simulink model "Vorlage_Gesamtanlage"  (R2022a)
settings: Solver=ode5  StartTime=0.0  StopTime=200  FixedStep=0.01  MaxStep=1  MinStep=0.005  RelTol=1e-3  AbsTol=10  EnableMultiTasking=on
values from neighbouring files (symbols this model uses):
  A = 5    [Parameter.m]
  Flaschengroesse = 10    [Parameter.m]
  I = 0.5    [Parameter.m]
  igetr = 1080    [Parameter.m]
  K = 8    [Parameter.m]
  MaxFlaschen = 25    [Parameter.m]
  MRK = 1    [Parameter.m]
  numA = 0    [Parameter.m]
  PassSilo1 = 1    [Parameter.m]
  PassSilo2 = 1    [Parameter.m]
  PHI = 0.001    [Parameter.m]
  Ra = 40    [Parameter.m]
  SizeSilo1 = 15    [Parameter.m]
  SizeSilo2 = 15    [Parameter.m]
  U = 24    [Parameter.m]
  v_band_abfuhr_set = 2    [Parameter.m]
  v_band_arbeit_set = 30    [Parameter.m]
  v_band_zufuhr_set = 10    [Parameter.m]
  v_umsetzer_greifer_set = 400    [Parameter.m]
  v_umsetzer_set = 80    [Parameter.m]
  v_ve1_set = 400    [Parameter.m]
  v_ve2_set = 400    [Parameter.m]
undefined symbols (not defined in the file or in its folder): Limits
libraries: simulink x94
(part 1 of 3)
settings Model: Creator=merz  LastModifiedBy=yufu
settings SolverCC: AutoScaleAbsTol=off  AlgebraicLoopSolver=TrustRegion
settings DataIOCC: LimitDataPoints=on  SaveFormat=Array  SignalLoggingSaveFormat=ModelDataLogs  ReturnWorkspaceOutputs=off  SignalLoggingName=sigsOut
settings OptimizationCC: ExpressionDepthLimit=2147483647  InitFltsAndDblsToZero=on  LifeSpan=inf
settings DebuggingCC: AlgebraicLoopMsg=none  SaveWithParameterizedLinksMsg=none  UnderspecifiedInitializationDetection=Classic  MergeDetectMultiDrivingBlocksExec=none  SignalResolutionControl=TryResolveAllWithWarning  MultiTaskDSMMsg=warning  MultiTaskCondExecSysMsg=none  FcnCallInpInsideContextMsg=warning  UnconnectedInputMsg=warning  UnconnectedOutputMsg=warning  UnconnectedLineMsg=warning  StateNameClashWarn=warning  SFUnexpectedBacktrackingDiag=warning  SFNoUnconditionalDefaultTransitionDiag=warning  SFMachineParentedDataDiag=warning  ArithmeticOperatorsInVariantConditions=warning
settings HardwareCC: ProdBitPerPointer=32  ProdBitPerSizeT=32  ProdBitPerPtrDiffT=32  ProdLargestAtomicFloat=None  ProdIntDivRoundTo=Undefined  ProdEndianess=Unspecified  ProdWordSize=32  ProdHWDeviceType=32-bit Generic  TargetUnknown=on
settings ModelReferenceCC: PropagateSignalLabelsOutOfModel=off
settings SFSimCC: SimUseLocalCustomCode=off  SimParseCustomCode=off  CustomCodeUndefinedFunction=UseInterfaceOnly
settings RTWCC: RTWUseLocalCustomCode=off
settings CodeAppCC: StateflowObjectComments=on
settings GRTTargetCC: TargetFcnLib=ansi_tfl_tmw.mat  TargetLangStandard=C89/C90 (ANSI)  ModelReferenceCompliant=off  CombineOutputUpdateFcns=off  MatFileLogging=off  GRTInterface=on
settings ConfigComp: CovMetricSettings=dw  CovSaveCumulativeToWorkspaceVar=on  CovSaveSingleToWorkspaceVar=on  CovExternalEMLEnable=off  CovSFcnEnable=off

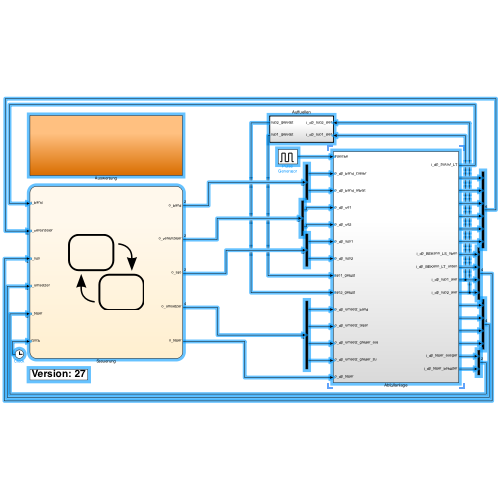
[thumbnail: Simulink's stored preview of the top-level diagram]
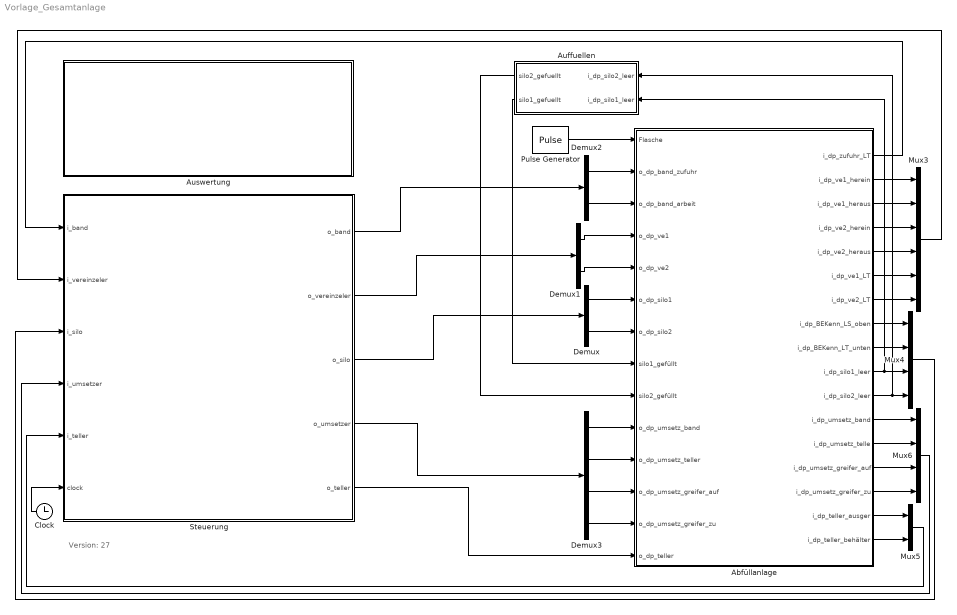
== system Vorlage_Gesamtanlage ==
  note: Version: 27
  Abfüllanlage : Subsystem
  Auffuellen : Subsystem  TreatAsAtomicUnit=on
  Auswertung : Subsystem
  Clock : Clock
  Demux : Demux  Outputs=2
      settings: DisplayOption=none
  Demux1 : Demux  Outputs=2
      settings: DisplayOption=none
  Demux2 : Demux  Outputs=2
      settings: DisplayOption=none
  Demux3 : Demux
      settings: DisplayOption=none
  Mux3 : Mux  Inputs=6
  Mux4 : Mux
  Mux5 : Mux  Inputs=2
  Mux6 : Mux
  Pulse Generator : DiscretePulseGenerator  PulseType=Time based  Period=5  PulseWidth=10  PhaseDelay=2
  Steuerung : Stateflow chart  TreatAsAtomicUnit=on
  wires:
  Steuerung/1(o_band) -> Demux2/1
  Steuerung/4(o_umsetzer) -> Demux3/1
  Steuerung/3(o_silo) -> Demux/1
  Steuerung/2(o_vereinzeler) -> Demux1/1
  Abfüllanlage/5(i_dp_ve2_heraus) -> Mux3/4
  Abfüllanlage/6(i_dp_ve1_LT) -> Mux3/5
  Abfüllanlage/7(i_dp_ve2_LT) -> Mux3/6
  Mux3/1 -> Steuerung/2(i_vereinzeler)
  Abfüllanlage/11(i_dp_silo2_leer) -> Auffuellen/1(i_dp_silo2_leer), Mux4/4
  Abfüllanlage/10(i_dp_silo1_leer) -> Mux4/3, Auffuellen/2(i_dp_silo1_leer)
  Abfüllanlage/8(i_dp_BEKenn_LS_oben) -> Mux4/1
  Abfüllanlage/16(i_dp_teller_ausger) -> Mux5/1
  Abfüllanlage/17(i_dp_teller_behälter) -> Mux5/2
  Mux5/1 -> Steuerung/5(i_teller)
  Abfüllanlage/1(i_dp_zufuhr_LT) -> Steuerung/1(i_band)
  Mux6/1 -> Steuerung/4(i_umsetzer)
  Demux/1 -> Abfüllanlage/6(o_dp_silo1)
  Demux/2 -> Abfüllanlage/7(o_dp_silo2)
  Demux1/1 -> Abfüllanlage/4(o_dp_ve1)
  Demux1/2 -> Abfüllanlage/5(o_dp_ve2)
  Demux2/1 -> Abfüllanlage/2(o_dp_band_zufuhr)
  Demux2/2 -> Abfüllanlage/3(o_dp_band_arbeit)
  Pulse Generator/1 -> Abfüllanlage/1(Flasche)
  Mux4/1 -> Steuerung/3(i_silo)
  Abfüllanlage/3(i_dp_ve1_heraus) -> Mux3/2
  Abfüllanlage/2(i_dp_ve1_herein) -> Mux3/1
  Abfüllanlage/4(i_dp_ve2_herein) -> Mux3/3
  Auffuellen/2(silo1_gefuellt) -> Abfüllanlage/8(silo1_gefüllt)
  Auffuellen/1(silo2_gefuellt) -> Abfüllanlage/9(silo2_gefüllt)
  Abfüllanlage/12(i_dp_umsetz_band) -> Mux6/1
  Abfüllanlage/13(i_dp_umsetz_telle) -> Mux6/2
  Abfüllanlage/14(i_dp_umsetz_greifer_auf) -> Mux6/3
  Abfüllanlage/15(i_dp_umsetz_greifer_zu) -> Mux6/4
  Demux3/1 -> Abfüllanlage/10(o_dp_umsetz_band)
  Demux3/2 -> Abfüllanlage/11(o_dp_umsetz_teller)
  Demux3/3 -> Abfüllanlage/12(o_dp_umsetz_greifer_auf)
  Demux3/4 -> Abfüllanlage/13(o_dp_umsetz_greifer_zu)
  Steuerung/5(o_teller) -> Abfüllanlage/14(o_dp_teller)
  Clock/1 -> Steuerung/6(clock)
  Abfüllanlage/9(i_dp_BEKenn_LT_unten) -> Mux4/2

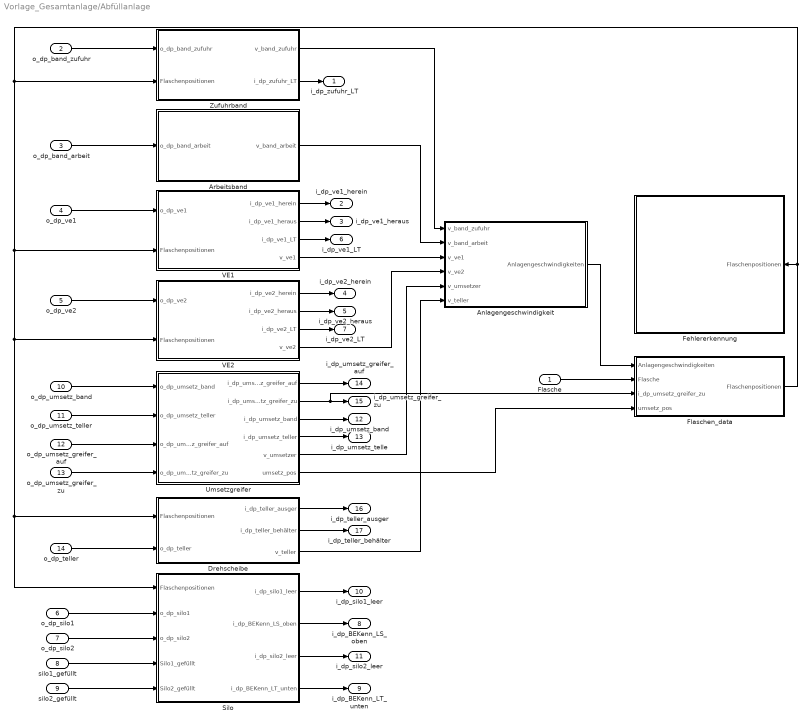
== system Vorlage_Gesamtanlage/Abfüllanlage ==
  Flasche : Inport
  o_dp_band_zufuhr : Inport  Port=2  OutDataTypeStr=double
  o_dp_band_arbeit : Inport  Port=3  OutDataTypeStr=double
  o_dp_ve1 : Inport  Port=4  OutDataTypeStr=double
  o_dp_ve2 : Inport  Port=5  OutDataTypeStr=double
  o_dp_silo1 : Inport  Port=6  OutDataTypeStr=double
  o_dp_silo2 : Inport  Port=7  OutDataTypeStr=double
  silo1_gefüllt : Inport  Port=8  OutDataTypeStr=double
  silo2_gefüllt : Inport  Port=9  OutDataTypeStr=double
  o_dp_umsetz_band : Inport  Port=10  OutDataTypeStr=double
  o_dp_umsetz_teller : Inport  Port=11  OutDataTypeStr=double
  o_dp_umsetz_greifer_auf : Inport  Port=12  OutDataTypeStr=double
  o_dp_umsetz_greifer_zu : Inport  Port=13  OutDataTypeStr=double
  o_dp_teller : Inport  Port=14  OutDataTypeStr=double
  Anlagengeschwindigkeit : Subsystem
  Arbeitsband : Subsystem
  Drehscheibe : Subsystem
  Fehlererkennung : Subsystem
  Flaschen_data : Subsystem
  Silo : Subsystem
  Umsetzgreifer : Subsystem
  VE1 : Subsystem
  VE2 : Subsystem
  Zufuhrband : Subsystem
  i_dp_zufuhr_LT : Outport  OutDataTypeStr=boolean
  i_dp_ve1_herein : Outport  Port=2  OutDataTypeStr=boolean
  i_dp_ve1_heraus : Outport  Port=3  OutDataTypeStr=boolean
  i_dp_ve2_herein : Outport  Port=4  OutDataTypeStr=boolean
  i_dp_ve2_heraus : Outport  Port=5  OutDataTypeStr=boolean
  i_dp_ve1_LT : Outport  Port=6  OutDataTypeStr=boolean
  i_dp_ve2_LT : Outport  Port=7  OutDataTypeStr=boolean
  i_dp_BEKenn_LS_oben : Outport  Port=8  OutDataTypeStr=boolean
  i_dp_BEKenn_LT_unten : Outport  Port=9  OutDataTypeStr=boolean
  i_dp_silo1_leer : Outport  Port=10  OutDataTypeStr=boolean
  i_dp_silo2_leer : Outport  Port=11  OutDataTypeStr=boolean
  i_dp_umsetz_band : Outport  Port=12  OutDataTypeStr=boolean
  i_dp_umsetz_telle : Outport  Port=13  OutDataTypeStr=boolean
  i_dp_umsetz_greifer_auf : Outport  Port=14  OutDataTypeStr=boolean
  i_dp_umsetz_greifer_zu : Outport  Port=15  OutDataTypeStr=boolean
  i_dp_teller_ausger : Outport  Port=16  OutDataTypeStr=boolean
  i_dp_teller_behälter : Outport  Port=17  OutDataTypeStr=boolean
  wires:
  Zufuhrband/1(v_band_zufuhr) -> Anlagengeschwindigkeit/1(v_band_zufuhr)
  VE1/4(v_ve1) -> Anlagengeschwindigkeit/3(v_ve1)
  Umsetzgreifer/5(v_umsetzer) -> Anlagengeschwindigkeit/5(v_umsetzer)
  Drehscheibe/3(v_teller) -> Anlagengeschwindigkeit/6(v_teller)
  Flaschen_data/1(Flaschenpositionen) -> Zufuhrband/2(Flaschenpositionen), VE1/2(Flaschenpositionen), VE2/2(Flaschenpositionen), Silo/1(Flaschenpositionen), Drehscheibe/1(Flaschenpositionen), Fehlererkennung/1(Flaschenpositionen)
  o_dp_band_zufuhr/1 -> Zufuhrband/1(o_dp_band_zufuhr)
  Zufuhrband/2(i_dp_zufuhr_LT) -> i_dp_zufuhr_LT/1
  o_dp_band_arbeit/1 -> Arbeitsband/1(o_dp_band_arbeit)
  VE1/1(i_dp_ve1_herein) -> i_dp_ve1_herein/1
  o_dp_ve1/1 -> VE1/1(o_dp_ve1)
  Silo/1(i_dp_silo1_leer) -> i_dp_silo1_leer/1
  VE1/2(i_dp_ve1_heraus) -> i_dp_ve1_heraus/1
  Silo/2(i_dp_BEKenn_LS_oben) -> i_dp_BEKenn_LS_oben/1
  VE1/3(i_dp_ve1_LT) -> i_dp_ve1_LT/1
  Silo/3(i_dp_silo2_leer) -> i_dp_silo2_leer/1
  Silo/4(i_dp_BEKenn_LT_unten) -> i_dp_BEKenn_LT_unten/1
  Umsetzgreifer/1(i_dp_umsetz_greifer_auf) -> i_dp_umsetz_greifer_auf/1
  o_dp_umsetz_band/1 -> Umsetzgreifer/1(o_dp_umsetz_band)
  o_dp_umsetz_teller/1 -> Umsetzgreifer/2(o_dp_umsetz_teller)
  Umsetzgreifer/3(i_dp_umsetz_band) -> i_dp_umsetz_band/1
  o_dp_umsetz_greifer_auf/1 -> Umsetzgreifer/3(o_dp_umsetz_greifer_auf)
  Umsetzgreifer/4(i_dp_umsetz_teller) -> i_dp_umsetz_telle/1
  o_dp_umsetz_greifer_zu/1 -> Umsetzgreifer/4(o_dp_umsetz_greifer_zu)
  Drehscheibe/1(i_dp_teller_ausger) -> i_dp_teller_ausger/1
  o_dp_teller/1 -> Drehscheibe/2(o_dp_teller)
  Drehscheibe/2(i_dp_teller_behälter) -> i_dp_teller_behälter/1
  o_dp_silo1/1 -> Silo/2(o_dp_silo1)
  o_dp_silo2/1 -> Silo/3(o_dp_silo2)
  silo2_gefüllt/1 -> Silo/5(Silo2_gefüllt)
  silo1_gefüllt/1 -> Silo/4(Silo1_gefüllt)
  Flasche/1 -> Flaschen_data/2(Flasche)
  Anlagengeschwindigkeit/1(Anlagengeschwindigkeiten) -> Flaschen_data/1(Anlagengeschwindigkeiten)
  VE2/2(i_dp_ve2_heraus) -> i_dp_ve2_heraus/1
  VE2/1(i_dp_ve2_herein) -> i_dp_ve2_herein/1
  VE2/3(i_dp_ve2_LT) -> i_dp_ve2_LT/1
  VE2/4(v_ve2) -> Anlagengeschwindigkeit/4(v_ve2)
  o_dp_ve2/1 -> VE2/1(o_dp_ve2)
  Umsetzgreifer/2(i_dp_umsetz_greifer_zu) -> i_dp_umsetz_greifer_zu/1, Flaschen_data/3(i_dp_umsetz_greifer_zu)
  Arbeitsband/1(v_band_arbeit) -> Anlagengeschwindigkeit/2(v_band_arbeit)
  Umsetzgreifer/6(umsetz_pos) -> Flaschen_data/4(umsetz_pos)

== system Vorlage_Gesamtanlage/Auffuellen ==
  i_dp_silo2_leer : Inport
  i_dp_silo1_leer : Inport  Port=2
  Data Type Conversion : DataTypeConversion  OutDataTypeStr=double  SaturateOnIntegerOverflow=off  RndMeth=Floor
  Data Type Conversion1 : DataTypeConversion  OutDataTypeStr=double  SaturateOnIntegerOverflow=off  RndMeth=Floor
  Transport Delay : TransportDelay  DelayTime=10
  Transport Delay1 : TransportDelay  DelayTime=10
  silo2_gefuellt : Outport
  silo1_gefuellt : Outport  Port=2
  wires:
  i_dp_silo1_leer/1 -> Data Type Conversion/1
  Transport Delay/1 -> silo1_gefuellt/1
  i_dp_silo2_leer/1 -> Data Type Conversion1/1
  Transport Delay1/1 -> silo2_gefuellt/1
  Data Type Conversion/1 -> Transport Delay/1
  Data Type Conversion1/1 -> Transport Delay1/1

== system Vorlage_Gesamtanlage/Auswertung ==
  Arbeitsband : Subsystem
  Drehscheibe : Subsystem
  Flaschen_data : Subsystem
  Gesamt : Subsystem
  Silo : Subsystem
  Umsetzgreifer : Subsystem
  Vereinzelner 1 : Subsystem
  Vereinzelner 2 : Subsystem
  Zufuhrband : Subsystem

== system Vorlage_Gesamtanlage/Abfüllanlage/Anlagengeschwindigkeit ==
  v_band_zufuhr : Inport
  v_band_arbeit : Inport  Port=2
  v_ve1 : Inport  Port=3
  v_ve2 : Inport  Port=4
  v_umsetzer : Inport  Port=5
  v_teller : Inport  Port=6
  Gain : Gain  Gain=3  SaturateOnIntegerOverflow=on  OutDataTypeStr=Inherit: Same as input  ParamDataTypeStr=Inherit: Same as input
  Mux : Mux  Inputs=10
  Wartestellung : Constant  Value=0
  v_band_abfuhr : Constant  Value=v_band_abfuhr_set
  Anlagengeschwindigkeiten : Outport
  wires:
  v_band_arbeit/1 -> Gain/1, Mux/3
  v_umsetzer/1 -> Mux/8, Mux/6
  Mux/1 -> Anlagengeschwindigkeiten/1
  v_band_abfuhr/1 -> Mux/10
  v_ve2/1 -> Mux/9
  v_teller/1 -> Mux/7
  Gain/1 -> Mux/5
  v_ve1/1 -> Mux/4
  v_band_zufuhr/1 -> Mux/2
  Wartestellung/1 -> Mux/1

== system Vorlage_Gesamtanlage/Abfüllanlage/Arbeitsband ==
  o_dp_band_arbeit : Inport
  Gain : Gain  Gain=v_band_arbeit_set  OutDataTypeStr=Inherit: Inherit via back propagation  SaturateOnIntegerOverflow=on  ParamDataTypeStr=Inherit: Same as input
  v_band_arbeit : Outport  OutDataTypeStr=double
  tag scope: o_dp_band_arbeit=global, v_band_arbeit=global
  wires:
  o_dp_band_arbeit/1 -> Gain/1, [o_dp_band_arbeit]  "o_dp_band_arbeit"
  Gain/1 -> v_band_arbeit/1, [v_band_arbeit]  "v_band_arbeit"

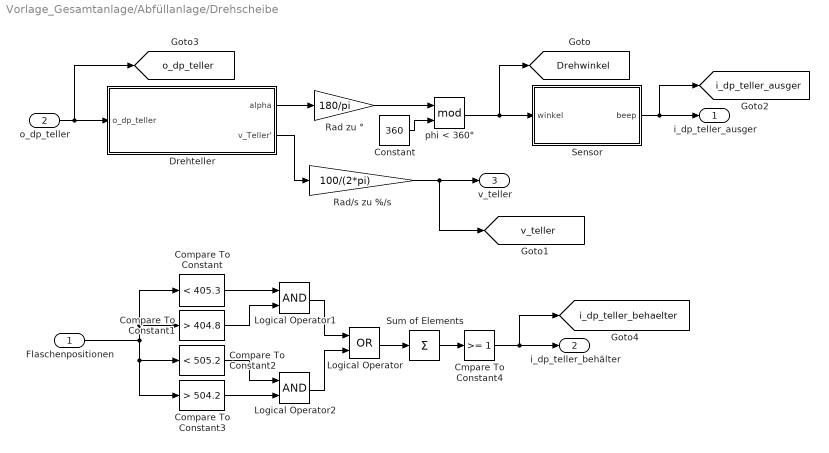
== system Vorlage_Gesamtanlage/Abfüllanlage/Drehscheibe ==
  Flaschenpositionen : Inport
  o_dp_teller : Inport  Port=2
  Cmpare To Constant4 : simulink/Logic and Bit Operations/Compare To Constant  relop=>=  const=1  OutDataTypeStr=boolean  ZeroCross=off
  Compare To Constant : simulink/Logic and Bit Operations/Compare To Constant  relop=<  const=405.3  OutDataTypeStr=boolean  ZeroCross=off
  Compare To Constant1 : simulink/Logic and Bit Operations/Compare To Constant  relop=>  const=404.8  OutDataTypeStr=boolean  ZeroCross=off
  Compare To Constant2 : simulink/Logic and Bit Operations/Compare To Constant  relop=<  const=505.2  OutDataTypeStr=boolean  ZeroCross=off
  Compare To Constant3 : simulink/Logic and Bit Operations/Compare To Constant  relop=>  const=504.2  OutDataTypeStr=boolean  ZeroCross=off
  Constant : Constant  Value=360
  Drehteller : Subsystem
  Logical Operator : Logic  Operator=OR  AllPortsSameDT=off  OutDataTypeStr=boolean
  Logical Operator1 : Logic  AllPortsSameDT=off  OutDataTypeStr=boolean
  Logical Operator2 : Logic  AllPortsSameDT=off  OutDataTypeStr=boolean
  Rad zu ° : Gain  Gain=180/pi  SaturateOnIntegerOverflow=on  OutDataTypeStr=Inherit: Same as input  ParamDataTypeStr=Inherit: Same as input
  Rad/s zu %/s : Gain  Gain=100/(2*pi)  SaturateOnIntegerOverflow=on  OutDataTypeStr=Inherit: Same as input  ParamDataTypeStr=Inherit: Same as input
  Sensor : Stateflow chart  TreatAsAtomicUnit=on
  Sum of Elements : Sum  Inputs=+
  phi < 360° : Math  Operator=mod  SignedPower=on
  i_dp_teller_ausger : Outport  OutDataTypeStr=boolean
  i_dp_teller_behälter : Outport  Port=2  OutDataTypeStr=boolean
  v_teller : Outport  Port=3  OutDataTypeStr=double
  tag scope: Drehwinkel=global, i_dp_teller_ausger=global, i_dp_teller_behaelter=global, o_dp_teller=global, v_teller=global
  wires:
  Sensor/1(beep) -> i_dp_teller_ausger/1, [i_dp_teller_ausger]
  phi < 360°/1 -> [Drehwinkel], Sensor/1(winkel)
  Rad zu °/1 -> phi < 360°/1
  Rad/s zu %/s/1 -> v_teller/1, [v_teller]
  Constant/1 -> phi < 360°/2
  o_dp_teller/1 -> Drehteller/1(o_dp_teller), [o_dp_teller]
  Drehteller/1(alpha) -> Rad zu °/1
  Drehteller/2(v_Teller') -> Rad/s zu %/s/1
  Logical Operator/1 -> Sum of Elements/1
  Compare To Constant/1 -> Logical Operator1/1
  Compare To Constant1/1 -> Logical Operator1/2
  Logical Operator1/1 -> Logical Operator/1
  Compare To Constant3/1 -> Logical Operator2/2
  Compare To Constant2/1 -> Logical Operator2/1
  Logical Operator2/1 -> Logical Operator/2
  Sum of Elements/1 -> Cmpare To Constant4/1
  Flaschenpositionen/1 -> Compare To Constant/1, Compare To Constant1/1, Compare To Constant3/1, Compare To Constant2/1
  Cmpare To Constant4/1 -> i_dp_teller_behälter/1, [i_dp_teller_behaelter]

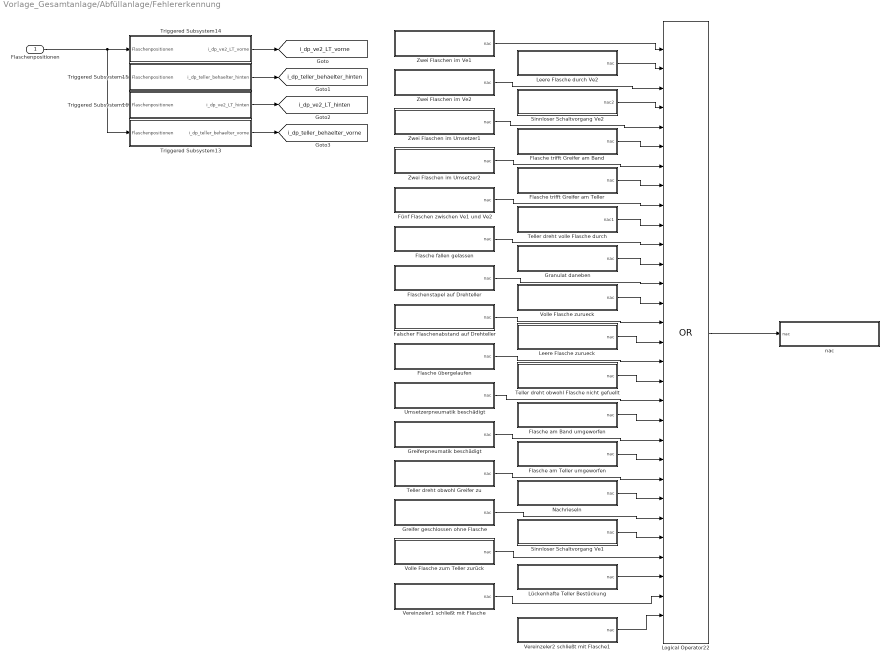
== system Vorlage_Gesamtanlage/Abfüllanlage/Fehlererkennung ==
  Flaschenpositionen : Inport
  Falscher Flaschenabstand auf Drehteller : Subsystem
  Flasche am Band umgeworfen : Subsystem
  Flasche am Teller umgeworfen : Subsystem
  Flasche fallen gelassen : Subsystem
  Flasche trifft Greifer am Band : Subsystem
  Flasche trifft Greifer am Teller : Subsystem
  Flasche übergelaufen : Subsystem
  Flaschenstapel auf Drehteller : Subsystem
  Fünf Flaschen zwischen Ve1 und Ve2 : Subsystem
  Granulat daneben : Subsystem
  Greifer geschlossen ohne Flasche : Subsystem
  Greiferpneumatik beschädigt : Subsystem
  Leere Flasche durch Ve2 : Subsystem
  Leere Flasche zurueck : Subsystem
  Logical Operator22 : Logic  Operator=OR  Inputs=30  AllPortsSameDT=off  OutDataTypeStr=boolean
  Lückenhafte Teller Bestückung : Subsystem
  Nachrieseln : Subsystem
  Sinnloser Schaltvorgang Ve1 : Subsystem
  Sinnloser Schaltvorgang Ve2 : Subsystem
  Teller dreht obwohl Flasche nicht gefuellt : Subsystem
  Teller dreht obwohl Greifer zu : Subsystem
  Teller dreht volle Flasche durch : Subsystem
  Triggered Subsystem13 : Subsystem  TreatAsAtomicUnit=on
  Triggered Subsystem14 : Subsystem  TreatAsAtomicUnit=on
  Triggered Subsystem15 : Subsystem  TreatAsAtomicUnit=on
  Triggered Subsystem16 : Subsystem  TreatAsAtomicUnit=on
  Umsetzerpneumatik beschädigt : Subsystem
  Vereinzeler1 schließt mit Flasche : Subsystem
  Vereinzeler2 schließt mit Flasche1 : Subsystem
  Volle Flasche zum Teller zurück : Subsystem
  Volle Flasche zurueck : Subsystem
  Zwei Flaschen im Umsetzer1 : Subsystem
  Zwei Flaschen im Umsetzer2 : Subsystem
  Zwei Flaschen im Ve1 : Subsystem
  Zwei Flaschen im Ve2 : Subsystem
  nac : Subsystem
  tag scope: i_dp_teller_behaelter_hinten=global, i_dp_teller_behaelter_vorne=global, i_dp_ve2_LT_hinten=global, i_dp_ve2_LT_vorne=global
  wires:
  Leere Flasche durch Ve2/1(nac) -> Logical Operator22/2
  Sinnloser Schaltvorgang Ve2/1(nac2) -> Logical Operator22/4
  Flasche trifft Greifer am Band/1(nac) -> Logical Operator22/6
  Flasche trifft Greifer am Teller/1(nac) -> Logical Operator22/8
  Teller dreht volle Flasche durch/1(nac1) -> Logical Operator22/10
  Granulat daneben/1(nac) -> Logical Operator22/12
  Flaschenstapel auf Drehteller/1(nac) -> Logical Operator22/13
  Volle Flasche zurueck/1(nac) -> Logical Operator22/14
  Flasche übergelaufen/1(nac) -> Logical Operator22/17
  Leere Flasche zurueck/1(nac) -> Logical Operator22/16
  Umsetzerpneumatik beschädigt/1(nac) -> Logical Operator22/19
  Teller dreht obwohl Flasche nicht gefuellt/1(nac) -> Logical Operator22/18
  Greiferpneumatik beschädigt/1(nac) -> Logical Operator22/21
  Flasche am Band umgeworfen/1(nac) -> Logical Operator22/20
  Flasche am Teller umgeworfen/1(nac) -> Logical Operator22/22
  Teller dreht obwohl Greifer zu/1(nac) -> Logical Operator22/23
  Falscher Flaschenabstand auf Drehteller/1(nac) -> Logical Operator22/15
  Flasche fallen gelassen/1(nac) -> Logical Operator22/11
  Fünf Flaschen zwischen Ve1 und Ve2/1(nac) -> Logical Operator22/9
  Zwei Flaschen im Umsetzer2/1(nac) -> Logical Operator22/7
  Zwei Flaschen im Umsetzer1/1(nac) -> Logical Operator22/5
  Zwei Flaschen im Ve2/1(nac) -> Logical Operator22/3
  Zwei Flaschen im Ve1/1(nac) -> Logical Operator22/1
  Triggered Subsystem14/1(i_dp_ve2_LT_vorne) -> [i_dp_ve2_LT_vorne]
  Triggered Subsystem15/1(i_dp_teller_behaelter_hinten) -> [i_dp_teller_behaelter_hinten]
  Triggered Subsystem16/1(i_dp_ve2_LT_hinten) -> [i_dp_ve2_LT_hinten]
  Triggered Subsystem13/1(i_dp_teller_behaelter_vorne) -> [i_dp_teller_behaelter_vorne]
  Flaschenpositionen/1 -> Triggered Subsystem14/1(Flaschenpositionen), Triggered Subsystem15/1(Flaschenpositionen), Triggered Subsystem16/1(Flaschenpositionen), Triggered Subsystem13/1(Flaschenpositionen)
  Nachrieseln/1(nac) -> Logical Operator22/24
  Greifer geschlossen ohne Flasche/1(nac) -> Logical Operator22/25
  Sinnloser Schaltvorgang Ve1/1(nac) -> Logical Operator22/26
  Volle Flasche zum Teller zurück/1(nac) -> Logical Operator22/27
  Lückenhafte Teller Bestückung/1(nac) -> Logical Operator22/28
  Vereinzeler1 schließt mit Flasche/1(nac) -> Logical Operator22/29
  Vereinzeler2 schließt mit Flasche1/1(nac) -> Logical Operator22/30
  Logical Operator22/1 -> nac/1(nac)

== system Vorlage_Gesamtanlage/Abfüllanlage/Flaschen_data ==
  Anlagengeschwindigkeiten : Inport
  Flasche : Inport  Port=2
  i_dp_umsetz_greifer_zu : Inport  Port=3
  umsetz_pos : Inport  Port=4
  Constant : Constant  Value=[0.01 101 201 205 305 405 505 605 610 inf]
  Flaschengeschwindigkeiten : Subsystem
  Flaschenstarter : Subsystem
  "v -> x" : Subsystem
  Flaschenpositionen : Outport
  tag scope: Flaschengeschwindigkeiten=global, Flaschenpositionen=global
  wires:
  Flasche/1 -> Flaschenstarter/2(Flasche)
  Flaschengeschwindigkeiten/1(Flaschengeschwindigkeiten) -> [Flaschengeschwindigkeiten], "v -> x"/1(Flaschengeschwindigkeiten)
  Anlagengeschwindigkeiten/1 -> Flaschengeschwindigkeiten/1(Anlagengeschwindigkeiten)
  Flaschenstarter/1(Flaschenpositionen mit Starter) -> Flaschengeschwindigkeiten/3(Flaschenpositionen)
  i_dp_umsetz_greifer_zu/1 -> Flaschengeschwindigkeiten/2(i_dp_umsetz_greifer_zu)
  umsetz_pos/1 -> Flaschengeschwindigkeiten/4(umsetz_pos)
  "v -> x"/1(Flaschenpositionen) -> Flaschenpositionen/1, [Flaschenpositionen], Flaschenstarter/1(Flaschenpositionen)
  Flaschengeschwindigkeiten/2(Anlagenpositionen) -> "v -> x"/2(Anlagenpositionen)
  Constant/1 -> "v -> x"/3(Anlagenlimits)

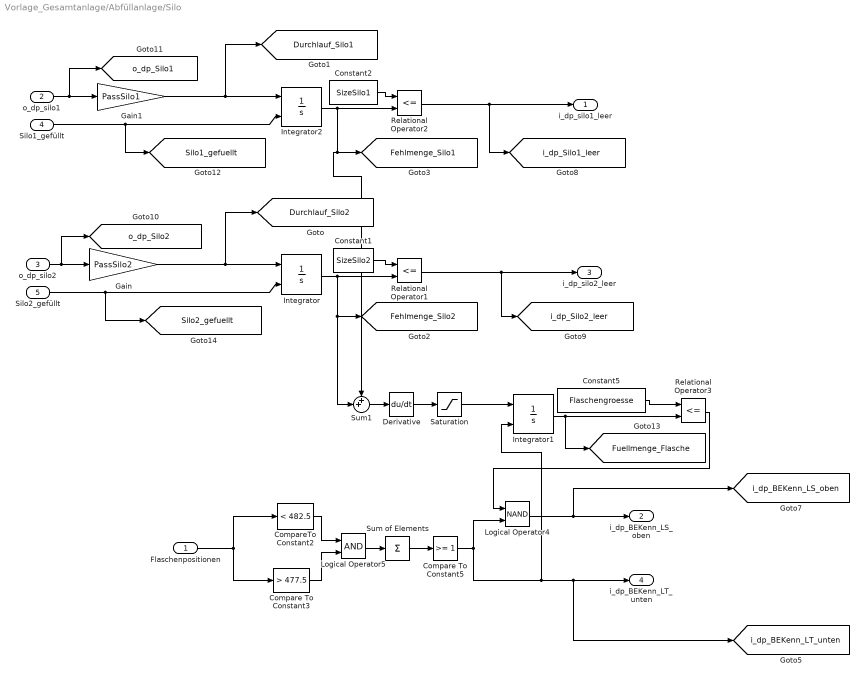
== system Vorlage_Gesamtanlage/Abfüllanlage/Silo ==
  Flaschenpositionen : Inport
  o_dp_silo1 : Inport  Port=2
  o_dp_silo2 : Inport  Port=3
  Silo1_gefüllt : Inport  Port=4
  Silo2_gefüllt : Inport  Port=5
  Compare To Constant3 : simulink/Logic and Bit Operations/Compare To Constant  relop=>  const=477.5  OutDataTypeStr=boolean  ZeroCross=off
  Compare To Constant5 : simulink/Logic and Bit Operations/Compare To Constant  relop=>=  const=1  OutDataTypeStr=boolean  ZeroCross=off
  CompareTo Constant2 : simulink/Logic and Bit Operations/Compare To Constant  relop=<  const=482.5  OutDataTypeStr=boolean  ZeroCross=off
  Constant1 : Constant  Value=SizeSilo2
  Constant2 : Constant  Value=SizeSilo1
  Constant5 : Constant  Value=Flaschengroesse
  Derivative : Derivative
  Gain : Gain  Gain=PassSilo2  SaturateOnIntegerOverflow=on  OutDataTypeStr=Inherit: Same as input  ParamDataTypeStr=Inherit: Same as input
  Gain1 : Gain  Gain=PassSilo1  SaturateOnIntegerOverflow=on  OutDataTypeStr=Inherit: Same as input  ParamDataTypeStr=Inherit: Same as input
  Integrator : Integrator  ExternalReset=rising  LimitOutput=on  UpperSaturationLimit=SizeSilo2  LowerSaturationLimit=0
  Integrator1 : Integrator  ExternalReset=falling  LimitOutput=on  LowerSaturationLimit=0
  Integrator2 : Integrator  ExternalReset=rising  LimitOutput=on  UpperSaturationLimit=SizeSilo1  LowerSaturationLimit=0
  Logical Operator4 : Logic  Operator=NAND  AllPortsSameDT=off  OutDataTypeStr=boolean
  Logical Operator5 : Logic  AllPortsSameDT=off  OutDataTypeStr=boolean
  Relational Operator1 : RelationalOperator  Operator=<=  InputSameDT=off
  Relational Operator2 : RelationalOperator  Operator=<=  InputSameDT=off
  Relational Operator3 : RelationalOperator  Operator=<=  InputSameDT=off
  Saturation : Saturate  UpperLimit=inf  LowerLimit=0
  Sum of Elements : Sum  Inputs=+
  Sum1 : Sum  Inputs=++|  SaturateOnIntegerOverflow=on
  i_dp_silo1_leer : Outport  OutDataTypeStr=boolean
  i_dp_BEKenn_LS_oben : Outport  Port=2  OutDataTypeStr=boolean
  i_dp_silo2_leer : Outport  Port=3  OutDataTypeStr=boolean
  i_dp_BEKenn_LT_unten : Outport  Port=4  OutDataTypeStr=boolean
  tag scope: Durchlauf_Silo1=global, Durchlauf_Silo2=global, Fehlmenge_Silo1=global, Fehlmenge_Silo2=global, Fuellmenge_Flasche=global, Silo1_gefuellt=global, Silo2_gefuellt=global, i_dp_BEKenn_LS_oben=global, i_dp_BEKenn_LT_unten=global, i_dp_Silo1_leer=global, i_dp_Silo2_leer=global, o_dp_Silo1=global, o_dp_Silo2=global
  wires:
  Constant2/1 -> Relational Operator2/1
  Relational Operator2/1 -> i_dp_silo1_leer/1, [i_dp_Silo1_leer]
  o_dp_silo1/1 -> Gain1/1, [o_dp_Silo1]
  Integrator2/1 -> Relational Operator2/2, [Fehlmenge_Silo1], Sum1/1
  o_dp_silo2/1 -> Gain/1, [o_dp_Silo2]
  Constant1/1 -> Relational Operator1/1
  Relational Operator1/1 -> i_dp_silo2_leer/1, [i_dp_Silo2_leer]
  Integrator/1 -> Relational Operator1/2, [Fehlmenge_Silo2], Sum1/2
  Silo1_gefüllt/1 -> Integrator2/2, [Silo1_gefuellt]
  Gain/1 -> Integrator/1, [Durchlauf_Silo2]
  Integrator1/1 -> [Fuellmenge_Flasche], Relational Operator3/2
  Constant5/1 -> Relational Operator3/1
  Sum1/1 -> Derivative/1
  Gain1/1 -> Integrator2/1, [Durchlauf_Silo1]
  Silo2_gefüllt/1 -> Integrator/2, [Silo2_gefuellt]
  CompareTo Constant2/1 -> Logical Operator5/1
  Compare To Constant3/1 -> Logical Operator5/2
  Sum of Elements/1 -> Compare To Constant5/1
  Logical Operator5/1 -> Sum of Elements/1
  Compare To Constant5/1 -> Logical Operator4/2, i_dp_BEKenn_LT_unten/1, [i_dp_BEKenn_LT_unten], Integrator1/2
  Logical Operator4/1 -> i_dp_BEKenn_LS_oben/1, [i_dp_BEKenn_LS_oben]
  Flaschenpositionen/1 -> CompareTo Constant2/1, Compare To Constant3/1
  Relational Operator3/1 -> Logical Operator4/1
  Derivative/1 -> Saturation/1
  Saturation/1 -> Integrator1/1

== system Vorlage_Gesamtanlage/Abfüllanlage/Umsetzgreifer ==
  o_dp_umsetz_band : Inport
  o_dp_umsetz_teller : Inport  Port=2
  o_dp_umsetz_greifer_auf : Inport  Port=3
  o_dp_umsetz_greifer_zu : Inport  Port=4
  Greifer : Subsystem
  Umsetzer : Subsystem
  i_dp_umsetz_greifer_auf : Outport  OutDataTypeStr=boolean
  i_dp_umsetz_greifer_zu : Outport  Port=2  OutDataTypeStr=boolean
  i_dp_umsetz_band : Outport  Port=3  OutDataTypeStr=boolean
  i_dp_umsetz_teller : Outport  Port=4  OutDataTypeStr=boolean
  v_umsetzer : Outport  Port=5  OutDataTypeStr=double
  umsetz_pos : Outport  Port=6  OutDataTypeStr=double
  wires:
  o_dp_umsetz_band/1 -> Umsetzer/1(o_dp_umsetz_band)
  o_dp_umsetz_teller/1 -> Umsetzer/2(o_dp_umsetz_teller)
  Umsetzer/1(v_umsetzer) -> v_umsetzer/1  "Geschwindigkeit"
  Umsetzer/2(i_dp_umsetz_teller) -> i_dp_umsetz_teller/1  "I_dp_umsetz_teller"
  Umsetzer/3(i_dp_umsetz_band) -> i_dp_umsetz_band/1  "I_dp_umsetz_band"
  o_dp_umsetz_greifer_auf/1 -> Greifer/1(o_dp_umsetz_greifer_auf)
  o_dp_umsetz_greifer_zu/1 -> Greifer/2(o_dp_umsetz_greifer_zu)
  Greifer/1(i_dp_umsetz_greifer_auf) -> i_dp_umsetz_greifer_auf/1
  Greifer/2(i_dp_umsetz_greifer_zu) -> i_dp_umsetz_greifer_zu/1
  Umsetzer/4(umsetz_pos) -> umsetz_pos/1

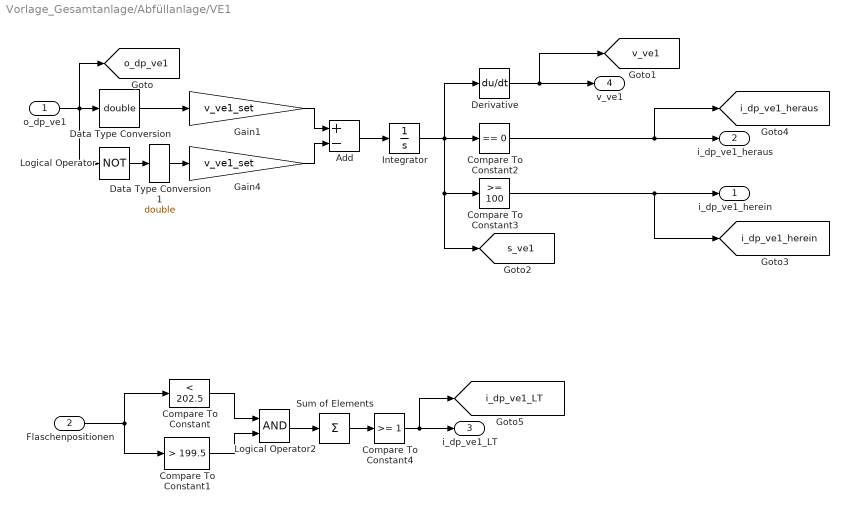
== system Vorlage_Gesamtanlage/Abfüllanlage/VE1 ==
  o_dp_ve1 : Inport
  Flaschenpositionen : Inport  Port=2
  Add : Sum  Inputs=+-
  Compare To Constant : simulink/Logic and Bit Operations/Compare To Constant  relop=<  const=202.5  OutDataTypeStr=boolean  ZeroCross=off
  Compare To Constant1 : simulink/Logic and Bit Operations/Compare To Constant  relop=>  const=199.5  OutDataTypeStr=boolean  ZeroCross=off
  Compare To Constant2 : simulink/Logic and Bit Operations/Compare To Constant  relop===  const=0  OutDataTypeStr=boolean  ZeroCross=off
  Compare To Constant3 : simulink/Logic and Bit Operations/Compare To Constant  relop=>=  const=100  OutDataTypeStr=boolean  ZeroCross=off
  Compare To Constant4 : simulink/Logic and Bit Operations/Compare To Constant  relop=>=  const=1  OutDataTypeStr=boolean  ZeroCross=off
  Data Type Conversion : DataTypeConversion  OutDataTypeStr=double  SaturateOnIntegerOverflow=off  RndMeth=Floor
  Data Type Conversion1 : DataTypeConversion  OutDataTypeStr=double  SaturateOnIntegerOverflow=off  RndMeth=Floor
  Derivative : Derivative
  Gain1 : Gain  Gain=v_ve1_set
  Gain4 : Gain  Gain=v_ve1_set
  Integrator : Integrator  LimitOutput=on  UpperSaturationLimit=100  LowerSaturationLimit=0
  Logical Operator : Logic  Operator=NOT  AllPortsSameDT=off  OutDataTypeStr=boolean
  Logical Operator2 : Logic  AllPortsSameDT=off  OutDataTypeStr=boolean
  Sum of Elements : Sum  Inputs=+
  i_dp_ve1_herein : Outport
  i_dp_ve1_heraus : Outport  Port=2
  i_dp_ve1_LT : Outport  Port=3  OutDataTypeStr=boolean
  v_ve1 : Outport  Port=4
  tag scope: i_dp_ve1_LT=global, i_dp_ve1_heraus=global, i_dp_ve1_herein=global, o_dp_ve1=global, s_ve1=global, v_ve1=global
  wires:
  Compare To Constant2/1 -> i_dp_ve1_heraus/1, [i_dp_ve1_heraus]
  o_dp_ve1/1 -> [o_dp_ve1], Data Type Conversion/1, Logical Operator/1
  Gain1/1 -> Add/1
  Gain4/1 -> Add/2
  Add/1 -> Integrator/1
  Integrator/1 -> Compare To Constant2/1, Derivative/1, Compare To Constant3/1, [s_ve1]
  Compare To Constant/1 -> Logical Operator2/1
  Compare To Constant1/1 -> Logical Operator2/2
  Logical Operator2/1 -> Sum of Elements/1
  Sum of Elements/1 -> Compare To Constant4/1
  Flaschenpositionen/1 -> Compare To Constant/1, Compare To Constant1/1
  Compare To Constant4/1 -> i_dp_ve1_LT/1, [i_dp_ve1_LT]
  Logical Operator/1 -> Data Type Conversion1/1
  Derivative/1 -> v_ve1/1, [v_ve1]
  Compare To Constant3/1 -> i_dp_ve1_herein/1, [i_dp_ve1_herein]
  Data Type Conversion/1 -> Gain1/1
  Data Type Conversion1/1 -> Gain4/1

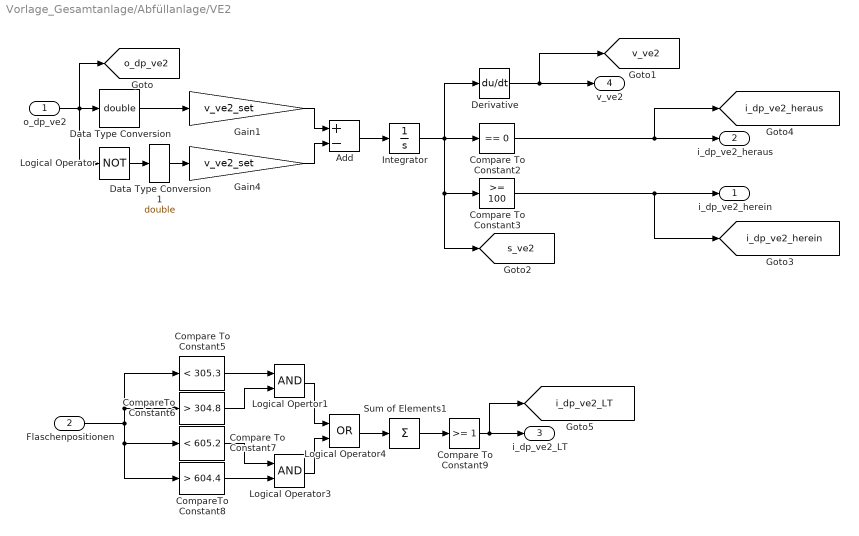
== system Vorlage_Gesamtanlage/Abfüllanlage/VE2 ==
  o_dp_ve2 : Inport
  Flaschenpositionen : Inport  Port=2
  Add : Sum  Inputs=+-
  Compare To Constant2 : simulink/Logic and Bit Operations/Compare To Constant  relop===  const=0  OutDataTypeStr=boolean  ZeroCross=off
  Compare To Constant3 : simulink/Logic and Bit Operations/Compare To Constant  relop=>=  const=100  OutDataTypeStr=boolean  ZeroCross=off
  Compare To Constant5 : simulink/Logic and Bit Operations/Compare To Constant  relop=<  const=305.3  OutDataTypeStr=boolean  ZeroCross=off
  Compare To Constant7 : simulink/Logic and Bit Operations/Compare To Constant  relop=<  const=605.2  OutDataTypeStr=boolean  ZeroCross=off
  Compare To Constant9 : simulink/Logic and Bit Operations/Compare To Constant  relop=>=  const=1  OutDataTypeStr=boolean  ZeroCross=off
  CompareTo Constant6 : simulink/Logic and Bit Operations/Compare To Constant  relop=>  const=304.8  OutDataTypeStr=boolean  ZeroCross=off
  CompareTo Constant8 : simulink/Logic and Bit Operations/Compare To Constant  relop=>  const=604.4  OutDataTypeStr=boolean  ZeroCross=off
  Data Type Conversion : DataTypeConversion  OutDataTypeStr=double  SaturateOnIntegerOverflow=off  RndMeth=Floor
  Data Type Conversion1 : DataTypeConversion  OutDataTypeStr=double  SaturateOnIntegerOverflow=off  RndMeth=Floor
  Derivative : Derivative
  Gain1 : Gain  Gain=v_ve2_set
  Gain4 : Gain  Gain=v_ve2_set
  Integrator : Integrator  LimitOutput=on  UpperSaturationLimit=100  LowerSaturationLimit=0
  Logical Operator : Logic  Operator=NOT  AllPortsSameDT=off  OutDataTypeStr=boolean
  Logical Operator3 : Logic  AllPortsSameDT=off  OutDataTypeStr=boolean
  Logical Operator4 : Logic  Operator=OR  AllPortsSameDT=off  OutDataTypeStr=boolean
  Logical Opertor1 : Logic  AllPortsSameDT=off  OutDataTypeStr=boolean
  Sum of Elements1 : Sum  Inputs=+
  i_dp_ve2_herein : Outport  OutDataTypeStr=boolean
  i_dp_ve2_heraus : Outport  Port=2  OutDataTypeStr=boolean
  i_dp_ve2_LT : Outport  Port=3  OutDataTypeStr=boolean
  v_ve2 : Outport  Port=4
  tag scope: i_dp_ve2_LT=global, i_dp_ve2_heraus=global, i_dp_ve2_herein=global, o_dp_ve2=global, s_ve2=global, v_ve2=global
  wires:
  Compare To Constant3/1 -> [i_dp_ve2_herein], i_dp_ve2_herein/1
  Derivative/1 -> [v_ve2], v_ve2/1
  Logical Operator/1 -> Data Type Conversion1/1
  Integrator/1 -> [s_ve2], Compare To Constant3/1, Derivative/1, Compare To Constant2/1
  Add/1 -> Integrator/1
  Gain4/1 -> Add/2
  Gain1/1 -> Add/1
  o_dp_ve2/1 -> [o_dp_ve2], Logical Operator/1, Data Type Conversion/1
  Compare To Constant2/1 -> [i_dp_ve2_heraus], i_dp_ve2_heraus/1
  Logical Opertor1/1 -> Logical Operator4/1
  Logical Operator3/1 -> Logical Operator4/2
  Logical Operator4/1 -> Sum of Elements1/1
  Compare To Constant7/1 -> Logical Operator3/1
  CompareTo Constant8/1 -> Logical Operator3/2
  Sum of Elements1/1 -> Compare To Constant9/1
  Compare To Constant5/1 -> Logical Opertor1/1
  CompareTo Constant6/1 -> Logical Opertor1/2
  Compare To Constant9/1 -> i_dp_ve2_LT/1, [i_dp_ve2_LT]
  Flaschenpositionen/1 -> CompareTo Constant6/1, Compare To Constant5/1, Compare To Constant7/1, CompareTo Constant8/1
  Data Type Conversion/1 -> Gain1/1
  Data Type Conversion1/1 -> Gain4/1

== system Vorlage_Gesamtanlage/Abfüllanlage/Zufuhrband ==
  o_dp_band_zufuhr : Inport
  Flaschenpositionen : Inport  Port=2
  Compare To Constant : simulink/Logic and Bit Operations/Compare To Constant  relop=<  const=4  OutDataTypeStr=boolean  ZeroCross=off
  Compare To Constant1 : simulink/Logic and Bit Operations/Compare To Constant  relop=>  const=0  OutDataTypeStr=boolean  ZeroCross=off
  Compare To Constant2 : simulink/Logic and Bit Operations/Compare To Constant  relop=>=  const=1  OutDataTypeStr=boolean  ZeroCross=off
  Gain : Gain  Gain=v_band_zufuhr_set  SaturateOnIntegerOverflow=on  OutDataTypeStr=Inherit: Same as input  ParamDataTypeStr=Inherit: Same as input
  Logical Operator : Logic  AllPortsSameDT=off  OutDataTypeStr=boolean
  Sum of Elements : Sum  Inputs=+
  v_band_zufuhr : Outport  OutDataTypeStr=double
  i_dp_zufuhr_LT : Outport  Port=2  OutDataTypeStr=boolean
  tag scope: i_dp_zufuhr_LT=global, o_dp_band_zufuhr=global, v_band_zufuhr=global
  wires:
  o_dp_band_zufuhr/1 -> Gain/1, [o_dp_band_zufuhr]  "o_dp_band_zufuhr"
  Gain/1 -> v_band_zufuhr/1, [v_band_zufuhr]  "v_band_zufuhr"
  Flaschenpositionen/1 -> Compare To Constant/1, Compare To Constant1/1
  Compare To Constant/1 -> Logical Operator/1
  Compare To Constant1/1 -> Logical Operator/2
  Logical Operator/1 -> Sum of Elements/1
  Sum of Elements/1 -> Compare To Constant2/1
  Compare To Constant2/1 -> i_dp_zufuhr_LT/1, [i_dp_zufuhr_LT]  "i_dp_zufuhr_LT"

== system Vorlage_Gesamtanlage/Auswertung/Arbeitsband ==
  Arbeitsbandüberwachung : Scope  NumInputPorts=2
  wires:
  [o_dp_band_arbeit] -> Arbeitsbandüberwachung/1  "o_dp_band_arbeit"
  [v_band_arbeit] -> Arbeitsbandüberwachung/2  "v_band_arbeit"

== system Vorlage_Gesamtanlage/Auswertung/Drehscheibe ==
  Drehtellerauswertung : Scope  NumInputPorts=5
  wires:
  [Drehwinkel] -> Drehtellerauswertung/1  "Drehwinkel"
  [v_teller] -> Drehtellerauswertung/2  "v_teller"
  [i_dp_teller_ausger] -> Drehtellerauswertung/3  "i_dp_teller_ausger"
  [i_dp_teller_behaelter] -> Drehtellerauswertung/4  "i_dp_teller_behälter"
  [o_dp_teller] -> Drehtellerauswertung/5  "o_dp_teller"

== system Vorlage_Gesamtanlage/Auswertung/Flaschen_data ==
  Auswertung Flaschen_data : Scope  NumInputPorts=5
  wires:
  [Flaschengeschwindigkeiten] -> Auswertung Flaschen_data/3  "Flaschengeschwindigkeiten"
  [Flaschenanzahl] -> Auswertung Flaschen_data/2  "Flaschenanzahl"
  [Flaschenpositionen] -> Auswertung Flaschen_data/1  "Flaschenpositionen"
  [Anlagenposition] -> Auswertung Flaschen_data/5  "Anlagenposition"
  [Flaschenanlagengeschwindigkeiten] -> Auswertung Flaschen_data/4  "Flaschenanlagengeschwindigkeiten"

== system Vorlage_Gesamtanlage/Auswertung/Gesamt ==
  Flaschenpositionen : Subsystem
  Inputs : Subsystem
  Outputs : Subsystem

== system Vorlage_Gesamtanlage/Auswertung/Silo ==
  Gesamt : Subsystem
  Silo1 : Subsystem
  Silo2 : Subsystem

== system Vorlage_Gesamtanlage/Auswertung/Umsetzgreifer ==
  Gesamt : Subsystem
  Greifer : Subsystem
  Umsetzer : Subsystem

== system Vorlage_Gesamtanlage/Auswertung/Vereinzelner 1 ==
  Auswertung des Vereinzelner 1 : Scope  NumInputPorts=6
  wires:
  [v_ve1] -> Auswertung des Vereinzelner 1/1  "Geschwindigkeit des Vereinzelners"
  [s_ve1] -> Auswertung des Vereinzelner 1/2  "Öffnungsweg"
  [o_dp_ve1] -> Auswertung des Vereinzelner 1/3  "o_dp_ve1"
  [i_dp_ve1_herein] -> Auswertung des Vereinzelner 1/4  "i_dp_ve1_herein"
  [i_dp_ve1_heraus] -> Auswertung des Vereinzelner 1/5  "i_dp_ve1_heraus"
  [i_dp_ve1_LT] -> Auswertung des Vereinzelner 1/6  "i_dp_ve1_LT"

== system Vorlage_Gesamtanlage/Auswertung/Vereinzelner 2 ==
  Auswertung des Vereinzelner 2 : Scope  NumInputPorts=6
  wires:
  [i_dp_ve2_LT] -> Auswertung des Vereinzelner 2/6  "i_dp_ve2_LT"
  [i_dp_ve2_heraus] -> Auswertung des Vereinzelner 2/5  "i_dp_ve2_heraus"
  [i_dp_ve2_herein] -> Auswertung des Vereinzelner 2/4  "i_dp_ve2_herein"
  [o_dp_ve2] -> Auswertung des Vereinzelner 2/3  "o_dp_ve2"
  [s_ve2] -> Auswertung des Vereinzelner 2/2  "Öffnungsweg"
  [v_ve2] -> Auswertung des Vereinzelner 2/1  "Geschwindigkeit des Vereinzelners"

== system Vorlage_Gesamtanlage/Auswertung/Zufuhrband ==
  Zufuhrbandüberwachung : Scope  NumInputPorts=3
  wires:
  [o_dp_band_zufuhr] -> Zufuhrbandüberwachung/1  "o_dp_band_zufuhr"
  [v_band_zufuhr] -> Zufuhrbandüberwachung/2  "v_band_zufuhr"
  [i_dp_zufuhr_LT] -> Zufuhrbandüberwachung/3  "i_dp_zufuhr_LT"

== system Vorlage_Gesamtanlage/Abfüllanlage/Drehscheibe/Drehteller ==
  o_dp_teller : Inport
  A : Gain  Gain=-A/I  SaturateOnIntegerOverflow=on  OutDataTypeStr=Inherit: Same as input  ParamDataTypeStr=Inherit: Same as input
  A1 : Gain  Gain=-K^2*PHI^2*igetr^2/Ra/I  SaturateOnIntegerOverflow=on  OutDataTypeStr=Inherit: Same as input  ParamDataTypeStr=Inherit: Same as input
  Constant : Constant  Value=-MRK/I
  Dead Zone : DeadZone
  Gain : Gain  Gain=U  SaturateOnIntegerOverflow=on
  Gain1 : Gain  Gain=K*PHI*igetr/Ra/I  SaturateOnIntegerOverflow=on  OutDataTypeStr=Inherit: Same as input  ParamDataTypeStr=Inherit: Same as input
  Integrator : Integrator
  Integrator1 : Integrator
  Product : Product  SaturateOnIntegerOverflow=on  OutDataTypeStr=Inherit: Same as first input
  Sign : Signum  ZeroCross=off
  Sum : Sum  Inputs=++|  SaturateOnIntegerOverflow=on
  Sum1 : Sum  Inputs=++|  SaturateOnIntegerOverflow=on
  Sum2 : Sum  Inputs=++|  SaturateOnIntegerOverflow=on
  alpha : Outport  OutDataTypeStr=double
  v_Teller' : Outport  Port=2  OutDataTypeStr=double
  wires:
  Integrator/1 -> A/1, A1/1, Dead Zone/1, Integrator1/1, v_Teller'/1  "Winkelgeschwindigkeit"
  o_dp_teller/1 -> Gain/1
  Gain/1 -> Gain1/1  "Spannung"
  Gain1/1 -> Sum/2  "Spannungsanteil"
  A/1 -> Sum/1  "linearer Reibungsanteil"
  Sum/1 -> Sum1/2
  A1/1 -> Sum1/1  "Selbstbehinderung"
  Sum1/1 -> Sum2/2
  Product/1 -> Sum2/1  "konstanter Reibungsanteil"
  Constant/1 -> Product/1
  Sign/1 -> Product/2  "Drehung vorhanden"
  Sum2/1 -> Integrator/1  "Winkelbeschleunigung"
  Integrator1/1 -> alpha/1
  Dead Zone/1 -> Sign/1

== system Vorlage_Gesamtanlage/Abfüllanlage/Fehlererkennung/Falscher Flaschenabstand auf Drehteller ==
  CompareTo Constant10 : simulink/Logic and Bit Operations/Compare To Constant  relop=>  const=26  OutDataTypeStr=boolean  ZeroCross=off
  CompareTo Constant16 : simulink/Logic and Bit Operations/Compare To Constant  relop=>  const=1  OutDataTypeStr=boolean  ZeroCross=off
  CompareTo Constant9 : simulink/Logic and Bit Operations/Compare To Constant  relop=<  const=24  OutDataTypeStr=boolean  ZeroCross=off
  Data Type Conversion : DataTypeConversion  OutDataTypeStr=double  SaturateOnIntegerOverflow=off  RndMeth=Floor
  Data Type Conversion1 : DataTypeConversion  OutDataTypeStr=boolean  SaturateOnIntegerOverflow=off  RndMeth=Floor
  Falscher Flaschenabstand auf Drehteller : Assertion
  Interval Test9 : simulink/Logic and Bit Operations/Interval Test  IntervalClosedRight=off  uplimit=500  IntervalClosedLeft=on  lowlimit=410  OutDataTypeStr=boolean
  Logical Operator11 : Logic  Operator=OR  AllPortsSameDT=off  OutDataTypeStr=boolean
  Logical Operator12 : Logic  AllPortsSameDT=off  OutDataTypeStr=boolean
  Logical Operator13 : Logic  Operator=NOT  AllPortsSameDT=off  OutDataTypeStr=boolean
  MATLAB Fcn : MATLABFcn  MATLABFcn=circshift(u, 1)-u
  MATLAB Fcn1 : MATLABFcn  MATLABFcn=circshift(u, 1)
  Memory7 : Memory  InitialCondition=1
  Product : Product  RndMeth=Zero
  Sum of Elements12 : Sum  Inputs=+
  nac : Outport
  wires:
  MATLAB Fcn/1 -> CompareTo Constant9/1, CompareTo Constant10/1
  CompareTo Constant9/1 -> Logical Operator11/1
  CompareTo Constant10/1 -> Logical Operator11/2
  Logical Operator11/1 -> Logical Operator12/1
  Interval Test9/1 -> Data Type Conversion/1
  Logical Operator13/1 -> Memory7/1
  Logical Operator12/1 -> Logical Operator13/1, Sum of Elements12/1
  Data Type Conversion/1 -> MATLAB Fcn1/1, Product/2
  MATLAB Fcn1/1 -> Product/1
  Product/1 -> Data Type Conversion1/1
  Data Type Conversion1/1 -> Logical Operator12/2
  Memory7/1 -> Falscher Flaschenabstand auf Drehteller/1
  Sum of Elements12/1 -> CompareTo Constant16/1
  CompareTo Constant16/1 -> nac/1
  [Flaschenpositionen] -> MATLAB Fcn/1, Interval Test9/1

== system Vorlage_Gesamtanlage/Abfüllanlage/Fehlererkennung/Flasche am Band umgeworfen ==
  Flasche am Band umgeworfen : Assertion
  Logical Operator12 : Logic  Inputs=3  AllPortsSameDT=off  OutDataTypeStr=boolean
  Logical Operator15 : Logic  Operator=NOT  AllPortsSameDT=off  OutDataTypeStr=boolean
  Memory : Memory  InitialCondition=1  InheritSampleTime=on
  Rising Edge : Subsystem
  nac : Outport
  wires:
  Logical Operator15/1 -> Memory/1
  Logical Operator12/1 -> Logical Operator15/1, nac/1
  Memory/1 -> Flasche am Band umgeworfen/1
  Rising Edge/1(edge) -> Logical Operator12/3
  [i_dp_umsetz_band] -> Rising Edge/1(signal)
  [i_dp_ve2_LT_vorne] -> Logical Operator12/1
  [i_dp_umsetz_greifer_zu] -> Logical Operator12/2

== system Vorlage_Gesamtanlage/Abfüllanlage/Fehlererkennung/Flasche am Teller umgeworfen ==
  Flasche am Teller umgeworfen : Assertion
  Logical Operator1 : Logic  Inputs=3  AllPortsSameDT=off  OutDataTypeStr=boolean
  Logical Operator2 : Logic  Operator=NOT  AllPortsSameDT=off  OutDataTypeStr=boolean
  Memory1 : Memory  InitialCondition=1  InheritSampleTime=on
  Rising Edge : Subsystem
  nac : Outport
  wires:
  Logical Operator1/1 -> nac/1, Logical Operator2/1
  Logical Operator2/1 -> Memory1/1
  Memory1/1 -> Flasche am Teller umgeworfen/1
  Rising Edge/1(edge) -> Logical Operator1/3
  [i_dp_umsetz_teller] -> Rising Edge/1(signal)
  [i_dp_teller_behaelter_hinten] -> Logical Operator1/1
  [i_dp_umsetz_greifer_zu] -> Logical Operator1/2

== system Vorlage_Gesamtanlage/Abfüllanlage/Fehlererkennung/Flasche fallen gelassen ==
  CompareTo Constant5 : simulink/Logic and Bit Operations/Compare To Constant  relop=>  const=0  OutDataTypeStr=boolean  ZeroCross=off
  CompareTo Constant6 : simulink/Logic and Bit Operations/Compare To Constant  relop=>  const=0  OutDataTypeStr=boolean  ZeroCross=off
  Flasche fallen gelassen : Assertion
  Interval Test5 : simulink/Logic and Bit Operations/Interval Test  IntervalClosedRight=off  uplimit=390  IntervalClosedLeft=on  lowlimit=310  OutDataTypeStr=boolean
  Interval Test6 : simulink/Logic and Bit Operations/Interval Test  IntervalClosedRight=off  uplimit=590  IntervalClosedLeft=on  lowlimit=510  OutDataTypeStr=boolean
  Logical Operator5 : Logic  Operator=NOT  AllPortsSameDT=off  OutDataTypeStr=boolean
  Logical Operator6 : Logic  AllPortsSameDT=off  OutDataTypeStr=boolean
  Logical Operator7 : Logic  Operator=NOT  AllPortsSameDT=off  OutDataTypeStr=boolean
  Logical Operator8 : Logic  Operator=OR  AllPortsSameDT=off  OutDataTypeStr=boolean
  Memory1 : Memory  InitialCondition=1
  Sum of Elements5 : Sum  Inputs=+
  Sum of Elements6 : Sum  Inputs=+
  nac : Outport
  wires:
  Sum of Elements5/1 -> CompareTo Constant5/1
  Interval Test5/1 -> Sum of Elements5/1
  Logical Operator6/1 -> Logical Operator5/1, nac/1
  Interval Test6/1 -> Sum of Elements6/1
  Sum of Elements6/1 -> CompareTo Constant6/1
  CompareTo Constant5/1 -> Logical Operator8/1
  CompareTo Constant6/1 -> Logical Operator8/2
  Logical Operator8/1 -> Logical Operator6/1
  Memory1/1 -> Flasche fallen gelassen/1
  Logical Operator5/1 -> Memory1/1
  Logical Operator7/1 -> Logical Operator6/2
  [i_dp_umsetz_greifer_zu] -> Logical Operator7/1
  [Flaschenpositionen] -> Interval Test5/1, Interval Test6/1

== system Vorlage_Gesamtanlage/Abfüllanlage/Fehlererkennung/Flasche trifft Greifer am Band ==
  Flasche triff Greifer am Band : Assertion
  Logical Operator12 : Logic  Inputs=3  AllPortsSameDT=off  OutDataTypeStr=boolean
  Logical Operator15 : Logic  Operator=NOT  AllPortsSameDT=off  OutDataTypeStr=boolean
  Memory : Memory  InitialCondition=1  InheritSampleTime=on
  Rising Edge : Subsystem
  nac : Outport
  wires:
  Logical Operator12/1 -> nac/1, Logical Operator15/1
  Logical Operator15/1 -> Memory/1
  Memory/1 -> Flasche triff Greifer am Band/1
  Rising Edge/1(edge) -> Logical Operator12/3
  [i_dp_ve2_LT_vorne] -> Rising Edge/1(signal)
  [i_dp_umsetz_band] -> Logical Operator12/1
  [i_dp_umsetz_greifer_zu] -> Logical Operator12/2

== system Vorlage_Gesamtanlage/Abfüllanlage/Fehlererkennung/Flasche trifft Greifer am Teller ==
  Flasche triff Greifer am Teller : Assertion
  Logical Operator12 : Logic  Inputs=3  AllPortsSameDT=off  OutDataTypeStr=boolean
  Logical Operator15 : Logic  Operator=NOT  AllPortsSameDT=off  OutDataTypeStr=boolean
  Memory : Memory  InitialCondition=1  InheritSampleTime=on
  Rising Edge : Subsystem
  nac : Outport
  wires:
  Logical Operator15/1 -> Memory/1
  Logical Operator12/1 -> Logical Operator15/1, nac/1
  Memory/1 -> Flasche triff Greifer am Teller/1
  [i_dp_teller_behaelter_hinten] -> Rising Edge/1(signal)
  Rising Edge/1(edge) -> Logical Operator12/3
  [i_dp_umsetz_teller] -> Logical Operator12/1
  [i_dp_umsetz_greifer_zu] -> Logical Operator12/2

== system Vorlage_Gesamtanlage/Abfüllanlage/Fehlererkennung/Flasche übergelaufen ==
  CompareTo Constant14 : simulink/Logic and Bit Operations/Compare To Constant  relop=>  const=10.1  OutDataTypeStr=boolean  ZeroCross=off
  Flasche übergelaufen : Assertion
  Logical Operator21 : Logic  Operator=NOT  AllPortsSameDT=off  OutDataTypeStr=boolean
  Memory8 : Memory  InitialCondition=1
  nac : Outport
  wires:
  CompareTo Constant14/1 -> Logical Operator21/1, nac/1
  Logical Operator21/1 -> Memory8/1
  Memory8/1 -> Flasche übergelaufen/1
  [Fuellmenge_Flasche] -> CompareTo Constant14/1

== system Vorlage_Gesamtanlage/Abfüllanlage/Fehlererkennung/Flaschenstapel auf Drehteller ==
  CompareTo Constant7 : simulink/Logic and Bit Operations/Compare To Constant  relop=>  const=0  OutDataTypeStr=boolean  ZeroCross=off
  CompareTo Constant8 : simulink/Logic and Bit Operations/Compare To Constant  relop=>  const=0  OutDataTypeStr=boolean  ZeroCross=off
  Flaschenstapel auf Drehteller : Assertion
  Interval Test7 : simulink/Logic and Bit Operations/Interval Test  IntervalClosedRight=off  uplimit=405  IntervalClosedLeft=on  lowlimit=395  OutDataTypeStr=boolean
  Interval Test8 : simulink/Logic and Bit Operations/Interval Test  IntervalClosedRight=off  uplimit=505  IntervalClosedLeft=on  lowlimit=495  OutDataTypeStr=boolean
  Logical Operator10 : Logic  Operator=NOT  AllPortsSameDT=off  OutDataTypeStr=boolean
  Logical Operator9 : Logic  AllPortsSameDT=off  OutDataTypeStr=boolean
  Memory : Memory  InitialCondition=1
  Sum of Elements7 : Sum  Inputs=+
  Sum of Elements8 : Sum  Inputs=+
  nac : Outport
  wires:
  Sum of Elements7/1 -> CompareTo Constant7/1
  Interval Test7/1 -> Sum of Elements7/1
  Interval Test8/1 -> Sum of Elements8/1
  Sum of Elements8/1 -> CompareTo Constant8/1
  CompareTo Constant7/1 -> Logical Operator9/1
  CompareTo Constant8/1 -> Logical Operator9/2
  Logical Operator10/1 -> Memory/1
  Logical Operator9/1 -> Logical Operator10/1, nac/1
  Memory/1 -> Flaschenstapel auf Drehteller/1
  [Flaschenpositionen] -> Interval Test7/1, Interval Test8/1

== system Vorlage_Gesamtanlage/Abfüllanlage/Fehlererkennung/Fünf Flaschen zwischen Ve1 und Ve2 ==
  CompareTo Constant4 : simulink/Logic and Bit Operations/Compare To Constant  relop=>  const=4  OutDataTypeStr=boolean  ZeroCross=off
  Fuenf Flaschen zwischen VE1 und VE2 : Assertion
  Interval Test4 : simulink/Logic and Bit Operations/Interval Test  IntervalClosedRight=off  uplimit=600  IntervalClosedLeft=on  lowlimit=210  OutDataTypeStr=boolean
  Logical Operator4 : Logic  Operator=NOT  AllPortsSameDT=off  OutDataTypeStr=boolean
  Memory2 : Memory  InitialCondition=1
  Sum of Elements4 : Sum  Inputs=+
  nac : Outport
  wires:
  Sum of Elements4/1 -> CompareTo Constant4/1
  Interval Test4/1 -> Sum of Elements4/1
  Logical Operator4/1 -> Memory2/1
  CompareTo Constant4/1 -> Logical Operator4/1, nac/1
  Memory2/1 -> Fuenf Flaschen zwischen VE1 und VE2/1
  [Flaschenpositionen] -> Interval Test4/1

== system Vorlage_Gesamtanlage/Abfüllanlage/Fehlererkennung/Granulat daneben ==
  CompareTo Constant13 : simulink/Logic and Bit Operations/Compare To Constant  relop===  const=0  OutDataTypeStr=boolean  ZeroCross=off
  Granulat daneben : Assertion
  Logical Operator18 : Logic  Operator=NOT  AllPortsSameDT=off  OutDataTypeStr=boolean
  Logical Operator19 : Logic  AllPortsSameDT=off  OutDataTypeStr=boolean
  Logical Operator20 : Logic  Operator=OR  AllPortsSameDT=off  OutDataTypeStr=boolean
  Memory11 : Memory  InitialCondition=1
  nac : Outport
  wires:
  Logical Operator18/1 -> Memory11/1
  Logical Operator20/1 -> Logical Operator19/2
  CompareTo Constant13/1 -> Logical Operator19/1
  Logical Operator19/1 -> Logical Operator18/1, nac/1
  Memory11/1 -> Granulat daneben/1
  [o_dp_Silo1] -> Logical Operator20/1
  [o_dp_Silo2] -> Logical Operator20/2
  [i_dp_BEKenn_LT_unten] -> CompareTo Constant13/1
